simulink model "Avalon_Interface"  (R2015a)
settings: Solver=ode45  StartTime=0.0  StopTime=10.0  RelTol=1e-3
InitFcn:
  | %% DSPBuilder Start
  | alt_dspbuilder_update_model(bdroot)
  | %% DSPBuilder End
libraries: allblocks_alteradspbuilder2 x6
settings Model: Creator=nguye  LastModifiedBy=nguye

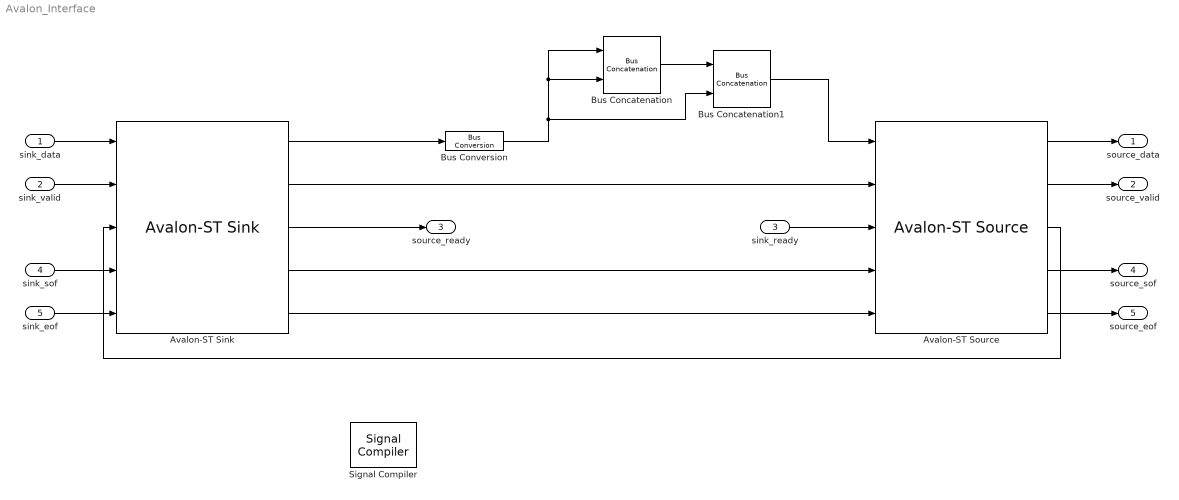
== system Avalon_Interface ==
  sink_data : Inport
  sink_valid : Inport  Port=2
  sink_ready : Inport  Port=3
  sink_sof : Inport  Port=4
  sink_eof : Inport  Port=5
  Avalon-ST Sink : allblocks_alteradspbuilder2/Avalon-ST Sink  iofile=G:\Project\PCIE_Display\custom_ip\tb_Avalon_Interface\Avalon%5FInterface_Avalon-ST+Sink_data.salt,G:\Project\PCIE_Display\custom_ip\tb_Avalon_Interface\Avalon%5FInterface_Avalon-ST+Sink_valid.salt,G:\Project\PCIE_Display\custom_ip\tb_Avalon_Interface\Avalon%5FInterface_Avalon-ST+Sink_ready.capture,G:\Project\PCIE_Display\custom_ip\tb_Avalon_Interface\Avalon%5FInterface_Avalon-ST+Sink_startofpacket.salt,G:\Project\PCIE_Display\custom_ip\tb_Avalon_Interface\Avalon%5FInterface_Avalon-ST+Sink_endofpacket.salt,  SpecifyClock=off  BusType=Unsigned Integer  bwl=24  bwr=0  symbolWidth=8  symbolsPerBeat=3  numOfChannels=0  numOfErrorDescriptors=0  endOfPacket=on  startOfPacket=on  empty=off  readyLatency=1  externalType=Inferred  PORTTYPE=Output
  Avalon-ST Source : allblocks_alteradspbuilder2/Avalon-ST Source  iofile=G:\Project\PCIE_Display\custom_ip\tb_Avalon_Interface\Avalon%5FInterface_Avalon-ST+Source_data.capture,G:\Project\PCIE_Display\custom_ip\tb_Avalon_Interface\Avalon%5FInterface_Avalon-ST+Source_valid.capture,G:\Project\PCIE_Display\custom_ip\tb_Avalon_Interface\Avalon%5FInterface_Avalon-ST+Source_ready.salt,G:\Project\PCIE_Display\custom_ip\tb_Avalon_Interface\Avalon%5FInterface_Avalon-ST+Source_startofpacket.capture,G:\Project\PCIE_Display\custom_ip\tb_Avalon_Interface\Avalon%5FInterface_Avalon-ST+Source_endofpacket.capture,  SpecifyClock=off  BusType=Unsigned Integer  bwl=24  bwr=0  symbolWidth=8  symbolsPerBeat=3  numOfChannels=0  numOfErrorDescriptors=0  endOfPacket=on  startOfPacket=on  empty=off  readyLatency=1  externalType=Inferred  PORTTYPE=Input
  Bus Concatenation : allblocks_alteradspbuilder2/Bus Concatenation  isSigned=off  awidth=8  bwidth=8  pipeline_display=0
  Bus Concatenation1 : allblocks_alteradspbuilder2/Bus Concatenation  isSigned=off  awidth=16  bwidth=8  pipeline_display=0
  Bus Conversion : allblocks_alteradspbuilder2/Bus Conversion  BusType=Unsigned Integer  ibwl=24  ibwr=1  bwl=8  bwr=1  bitToConnectToOutputLSB=0  round=off  saturate=off  pipeline_display=0
  Signal Compiler : allblocks_alteradspbuilder2/Signal Compiler  DeviceFamily=Cyclone IV GX  DeviceName=EP4CGX150DF31C7  DisableEarlyHDLGeneration=off  EnableSignalTap=off  SignalTapDepth=128  UseBoardBlock=off  StpUseDefaultClock=on  StpClock=Clock  ExportDir=C:\Users\nguye\OneDrive\Documents  MAX10_ProgrammingMode=Internal Flash (SDM) Single Boot
  source_data : Outport
  source_valid : Outport  Port=2
  source_ready : Outport  Port=3
  source_sof : Outport  Port=4
  source_eof : Outport  Port=5
  wires:
  Avalon-ST Sink/1 -> Bus Conversion/1
  sink_data/1 -> Avalon-ST Sink/1
  sink_valid/1 -> Avalon-ST Sink/2
  sink_eof/1 -> Avalon-ST Sink/5
  Avalon-ST Source/1 -> source_data/1
  Avalon-ST Source/2 -> source_valid/1
  Avalon-ST Source/4 -> source_sof/1
  Avalon-ST Source/5 -> source_eof/1
  sink_sof/1 -> Avalon-ST Sink/4
  Avalon-ST Sink/5 -> Avalon-ST Source/5
  Avalon-ST Sink/4 -> Avalon-ST Source/4
  Avalon-ST Sink/2 -> Avalon-ST Source/2
  Avalon-ST Sink/3 -> source_ready/1
  sink_ready/1 -> Avalon-ST Source/3
  Avalon-ST Source/3 -> Avalon-ST Sink/3
  Bus Conversion/1 -> Bus Concatenation/2, Bus Concatenation/1, Bus Concatenation1/2
  Bus Concatenation/1 -> Bus Concatenation1/1
  Bus Concatenation1/1 -> Avalon-ST Source/1
